simulink model "kinematic_sim"  (R2023a)
settings: Solver=FixedStepAuto  StartTime=0.0  StopTime=6  FixedStep=0.01  RelTol=1e-3
settings Model: Creator=arian  LastModifiedBy=arian

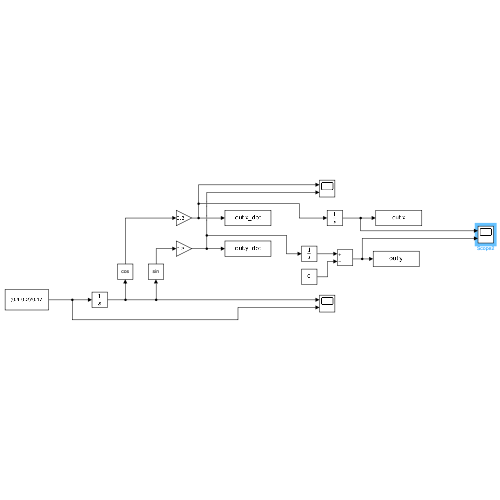
[thumbnail: Simulink's stored preview of the top-level diagram]
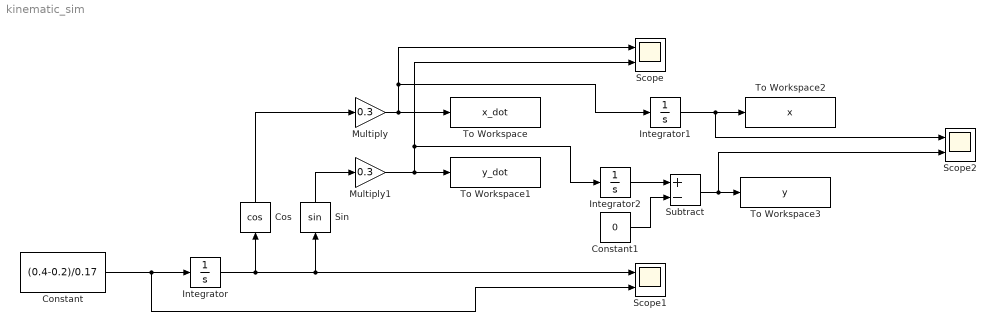
== system kinematic_sim ==
  Constant : Constant  Value=(0.4-0.2)/0.17
  Constant1 : Constant  Value=0
  Cos : Trigonometry  Operator=cos
  Integrator : Integrator
  Integrator1 : Integrator
  Integrator2 : Integrator
  Multiply : Gain  Gain=0.3
  Multiply1 : Gain  Gain=0.3
  Scope : Scope  NumInputPorts=2
  Scope1 : Scope  NumInputPorts=2
  Scope2 : Scope  NumInputPorts=2
  Sin : Trigonometry
  Subtract : Sum  Inputs=+-
  To Workspace : ToWorkspace  VariableName=x_dot  SampleTime=-1
      settings: Save2DSignal=2-D array (concatenate along first dimension)
  To Workspace1 : ToWorkspace  VariableName=y_dot  SampleTime=-1
      settings: Save2DSignal=2-D array (concatenate along first dimension)
  To Workspace2 : ToWorkspace  VariableName=x  SampleTime=-1
      settings: Save2DSignal=2-D array (concatenate along first dimension)
  To Workspace3 : ToWorkspace  VariableName=y  SampleTime=-1
      settings: Save2DSignal=2-D array (concatenate along first dimension)
  wires:
  Constant/1 -> Scope1/2, Integrator/1
  Integrator/1 -> Sin/1, Scope1/1, Cos/1
  Cos/1 -> Multiply/1
  Sin/1 -> Multiply1/1
  Multiply/1 -> To Workspace/1, Integrator1/1, Scope/1
  Multiply1/1 -> Integrator2/1, Scope/2, To Workspace1/1
  Integrator1/1 -> To Workspace2/1, Scope2/1
  Integrator2/1 -> Subtract/1
  Subtract/1 -> Scope2/2, To Workspace3/1
  Constant1/1 -> Subtract/2
